simulink model "MO_PHONG_MACH_BOOST"  (R2020a)
settings: Solver=VariableStepAuto  StartTime=0.0  StopTime=0.5  MaxStep=1e-4  RelTol=1e-3
values from neighbouring files (symbols this model uses):
  C = 7*Co_min_ripple    (= 0.000233333333333)    [Boost_Converter_Calc.m]    (also in TINH_TOAN_BO_DIEU_KHIEN_TYPE_III.m = 4.7e-05; boostControllerCalPID.m = 4.7e-05)
  Gc = kc*Gc1    [TINH_TOAN_BO_DIEU_KHIEN_TYPE_III.m]    (also in boostControllerCalPID.m)
  L = 0.9*Lmax    (= 1.3125e-05)    [Boost_Converter_Calc.m]    (also in TINH_TOAN_BO_DIEU_KHIEN_TYPE_III.m = 0.00012; boostControllerCalPID.m = 0.00012)
  R = Rmin    (= 15)    [Boost_Converter_Calc.m]    (also in TINH_TOAN_BO_DIEU_KHIEN_TYPE_III.m; boostControllerCalPID.m)
  Vo = 30    [Boost_Converter_Calc.m]    (also in TINH_TOAN_BO_DIEU_KHIEN_TYPE_III.m; boostControllerCalPID.m)
libraries: powerlib x9, powerlib_meascontrol x1
settings Model: Creator=Hello  LastModifiedBy=ngtuan
settings DataIOCC: ReturnWorkspaceOutputs=off
settings DebuggingCC: UnconnectedInputMsg=none  UnconnectedOutputMsg=none  UnconnectedLineMsg=none  ArithmeticOperatorsInVariantConditions=warning
settings SFSimCC: SimUseLocalCustomCode=off  CustomCodeUndefinedFunction=UseInterfaceOnly
settings RTWCC: RTWUseLocalCustomCode=off

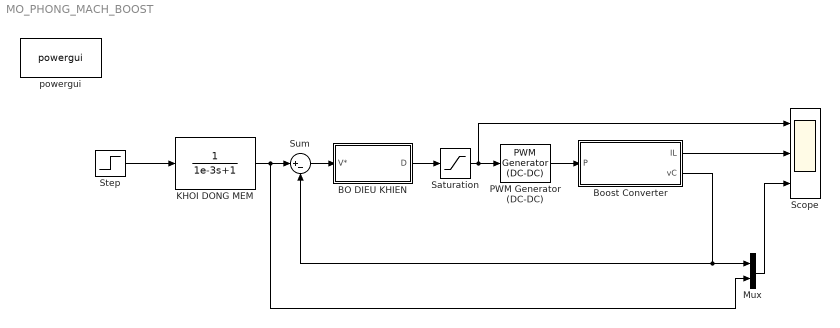
== system MO_PHONG_MACH_BOOST ==
  BO DIEU KHIEN : Subsystem
  Boost Converter : Subsystem
  KHOI DONG MEM : TransferFcn  Denominator=[1e-3 1]
  Mux : Mux  Inputs=2
  PWM Generator (DC-DC) : powerlib_meascontrol/Pulse & Signal Generators/PWM Generator (DC-DC)  Fsw=100000  Ts=0
  Saturation : Saturate  UpperLimit=1  LowerLimit=-1
  Scope : Scope  NumInputPorts=3
  Step : Step  Time=0.25  Before=20  After=Vo  SampleTime=0
  Sum : Sum  Inputs=|+-
  powergui : powerlib/powergui  Priority=1  SimulationMode=Continuous  SampleTime=50e-6  frequency=60  Iterations=50  frequencyindice=60  Pbase=100e6  ErrMax=1e-4  UnitsV=kV  UnitsW=MW  buscounter=0  FunctionMessages=off  echomessages=off  EnableUseOfTLC=off  CurrentSourceSwitches=off  DisableSnubberDevices=off  DisableRonSwitches=off  DisableVfSwitches=off  DisplayEquations=off  AutomaticDiscreteSolvers=off  SolverType=Tustin/Backward Euler (TBE)  Interpol=off  ExternalGateDelay=off  methode=off  Ts=100  x0status=blocks  SPID=on  SwTol=0  HookPort=off  NonlinearTolerance=1e-4  nMaxIteration=100  ContinueOnMaxIteration=off  RestoreLinks=warning  ResistiveCurrentMeasurement=off  Frange=[0:2:500]  Ylog=off  Xlog=on  ShowGrid=off  save=off  variable=ZData  structure=0  ZoomFFT=off  StartTime=0.0  cycles=1  DisplayStyle=1  fundamental=60  FreqAxis=off  MaxFrequency=1000  frequencyindicesteady=1  RmsSteady=1  display=off
  wires:
  PWM Generator (DC-DC)/1 -> Boost Converter/1(P)
  Step/1 -> KHOI DONG MEM/1
  Sum/1 -> BO DIEU KHIEN/1(V*)
  Mux/1 -> Scope/3
  KHOI DONG MEM/1 -> Mux/2, Sum/1
  Boost Converter/1(IL) -> Scope/2
  Saturation/1 -> Scope/1, PWM Generator (DC-DC)/1
  BO DIEU KHIEN/1(D) -> Saturation/1
  Boost Converter/2(vC) -> Sum/2, Mux/1

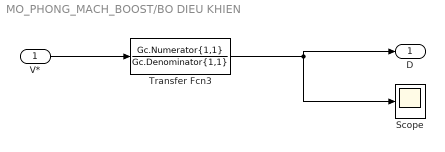
== system MO_PHONG_MACH_BOOST/BO DIEU KHIEN ==
  V* : Inport
  Scope : Scope
  Transfer Fcn3 : TransferFcn  Numerator=Gc.Numerator{1,1}  Denominator=Gc.Denominator{1,1}
  D : Outport  VectorParamsAs1DForOutWhenUnconnected=off
  wires:
  V*/1 -> Transfer Fcn3/1
  Transfer Fcn3/1 -> D/1, Scope/1

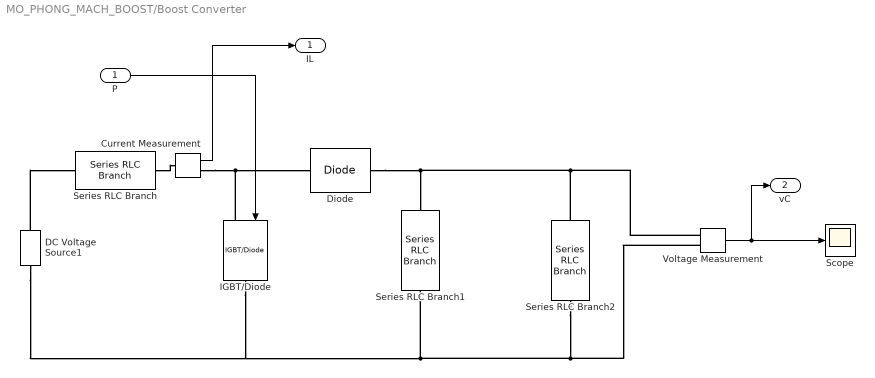
== system MO_PHONG_MACH_BOOST/Boost Converter ==
  P : Inport
  Current Measurement : powerlib/Measurements/Current Measurement  PhasorSimulation=off  OutputType=Complex  PSBequivalent=0
  DC Voltage Source1 : powerlib/Electrical Sources/DC Voltage Source  Amplitude=12  Measurements=None
  Diode : powerlib/Power Electronics/Diode  Ron=0.001  Lon=0  Vf=0  IC=0  UseSnubber=0  Rs=inf  Cs=inf  Measurements=off
  IGBT/Diode : powerlib/Power Electronics/IGBT//Diode  Ron=0.001  Rs=inf  Cs=inf  Measurements=off
  Scope : Scope
  Series RLC Branch : powerlib/Elements/Series RLC Branch  LConnTagsString=__new0  RConnTagsString=__new0  BranchType=L  Resistance=1  Inductance=L  SetiL0=off  InitialCurrent=0  Capacitance=1e-6  Setx0=off  InitialVoltage=0  Measurements=None
  Series RLC Branch1 : powerlib/Elements/Series RLC Branch  LConnTagsString=__new0  RConnTagsString=__new0  BranchType=C  Resistance=1  Inductance=1e-3  SetiL0=off  InitialCurrent=0  Capacitance=C  Setx0=on  InitialVoltage=12  Measurements=None
  Series RLC Branch2 : powerlib/Elements/Series RLC Branch  LConnTagsString=__new0  RConnTagsString=__new0  BranchType=R  Resistance=R  Inductance=1e-3  SetiL0=off  InitialCurrent=0  Capacitance=R  Setx0=off  InitialVoltage=0  Measurements=None
  Voltage Measurement : powerlib/Measurements/Voltage Measurement  PhasorSimulation=off  OutputType=Complex  PSBequivalent=0
  IL : Outport  VectorParamsAs1DForOutWhenUnconnected=off
  vC : Outport  Port=2  VectorParamsAs1DForOutWhenUnconnected=off
  wires:
  Current Measurement/1 -> IL/1
  Voltage Measurement/1 -> vC/1, Scope/1
  P/1 -> IGBT/Diode/1
  connections:
  DC Voltage Source1/RConn1 -- Series RLC Branch/LConn1
  IGBT/Diode/LConn1 -- Current Measurement/RConn1 -- Diode/LConn1
  Series RLC Branch2/LConn1 -- Voltage Measurement/LConn1 -- Series RLC Branch1/LConn1 -- Diode/RConn1
  Series RLC Branch2/RConn1 -- Voltage Measurement/LConn2 -- DC Voltage Source1/LConn1 -- IGBT/Diode/RConn1 -- Series RLC Branch1/RConn1
  Series RLC Branch/RConn1 -- Current Measurement/LConn1
